simulink library "FF_Library"  (R2024b)
settings: Solver=VariableStepAuto  StartTime=0.0  StopTime=10.0  RelTol=1e-3
undefined symbols (not defined in the file or in its folder): Slope1, Slope2
libraries: simulink x60
(part 4 of 4)

== system FF_Library/Memory/SAMPLEANDHOLD_RE/Functionality ==
  u : Inport
  E : Inport  Port=2
  R : Inport  Port=3
  IV : Inport  Port=4
  x_in : Inport  Port=5
  Data Type Duplicate : DataTypeDuplicate  NumInputPorts=3
  Signal Conversion : SignalConversion  ConversionOutput=Contiguous copy  OverrideOpt=off
  Signal Conversion1 : SignalConversion  ConversionOutput=Contiguous copy  OverrideOpt=off
  Switch : Switch  Criteria=u2 ~= 0  OutDataTypeStr=Inherit: Inherit via back propagation  SaturateOnIntegerOverflow=off
  Switch1 : Switch  Criteria=u2 ~= 0  OutDataTypeStr=Inherit: Inherit via back propagation  SaturateOnIntegerOverflow=off
  y : Outport
  x_out : Outport  Port=2
  wires:
  Switch/1 -> Data Type Duplicate/1, Signal Conversion1/1, Signal Conversion/1
  x_in/1 -> Data Type Duplicate/2, Switch1/3
  u/1 -> Switch1/1
  E/1 -> Switch1/2
  Switch1/1 -> Switch/3
  IV/1 -> Data Type Duplicate/3, Switch/1
  R/1 -> Switch/2
  Signal Conversion/1 -> y/1
  Signal Conversion1/1 -> x_out/1

== system FF_Library/Ctrl/PID/PID/Delay_Ext_Reset_IV ==
  u : Inport
  R : Inport  Port=2  OutDataTypeStr=boolean
  IV : Inport  Port=3
  Constant : Constant  Value=0  OutDataTypeStr=boolean
  Data Type Duplicate : DataTypeDuplicate  NumInputPorts=3
  OR : Logic  Operator=OR  OutDataTypeStr=boolean
  Switch2 : Switch  Criteria=u2 > Threshold  InputSameDT=off
      settings: AttributesFormatString=%<Criteria>
  Unit Delay : UnitDelay  SampleTime=-1  HasFrameUpgradeWarning=on
      settings: AttributesFormatString=%<InitialCondition>
  Unit Delay1 : UnitDelay  InitialCondition=1  SampleTime=-1  HasFrameUpgradeWarning=on
      settings: AttributesFormatString=%<InitialCondition>
  y : Outport
  wires:
  Switch2/1 -> y/1, Data Type Duplicate/1
  u/1 -> Unit Delay/1, Data Type Duplicate/3
  R/1 -> OR/1
  Constant/1 -> Unit Delay1/1
  Unit Delay/1 -> Switch2/3
  IV/1 -> Switch2/1, Data Type Duplicate/2
  Unit Delay1/1 -> OR/2
  OR/1 -> Switch2/2

== system FF_Library/Ctrl/PID/PID/Delay_Ext_Reset_IV1 ==
  u : Inport
  R : Inport  Port=2  OutDataTypeStr=boolean
  IV : Inport  Port=3
  Constant : Constant  Value=0  OutDataTypeStr=boolean
  Data Type Duplicate : DataTypeDuplicate  NumInputPorts=3
  OR : Logic  Operator=OR  OutDataTypeStr=boolean
  Switch2 : Switch  Criteria=u2 > Threshold  InputSameDT=off
      settings: AttributesFormatString=%<Criteria>
  Unit Delay : UnitDelay  SampleTime=-1  HasFrameUpgradeWarning=on
      settings: AttributesFormatString=%<InitialCondition>
  Unit Delay1 : UnitDelay  InitialCondition=1  SampleTime=-1  HasFrameUpgradeWarning=on
      settings: AttributesFormatString=%<InitialCondition>
  y : Outport
  wires:
  Switch2/1 -> y/1, Data Type Duplicate/1
  u/1 -> Unit Delay/1, Data Type Duplicate/3
  R/1 -> OR/1
  Constant/1 -> Unit Delay1/1
  Unit Delay/1 -> Switch2/3
  IV/1 -> Switch2/1, Data Type Duplicate/2
  Unit Delay1/1 -> OR/2
  OR/1 -> Switch2/2

== system FF_Library/Filter/HIGHPASST_RE/Functionality/DIV ==
  In1 : Inport
  In2 : Inport  Port=2
  Constant2 : Constant  Value=abs(MinRange)  OutDataTypeStr=Inherit: Inherit via back propagation
  Constant3 : Constant  Value=-abs(MinRange)  OutDataTypeStr=Inherit: Inherit via back propagation
  Constant7 : Constant  Value=0  OutDataTypeStr=Inherit: Inherit via back propagation
  Divide1 : Product  Inputs=*/  SaturateOnIntegerOverflow=on
  Max2 : MinMax  Function=max  Inputs=2
  Min : MinMax  Inputs=2
  Relational Operator : RelationalOperator  OutDataTypeStr=boolean  RndMeth=Simplest  InputSameDT=off
  Switch : Switch  Criteria=u2 > Threshold  InputSameDT=off
  Out1 : Outport
  wires:
  Constant3/1 -> Min/2
  Min/1 -> Switch/3
  Constant2/1 -> Max2/2
  In1/1 -> Divide1/1
  Divide1/1 -> Out1/1
  Relational Operator/1 -> Switch/2
  Switch/1 -> Divide1/2
  Constant7/1 -> Relational Operator/2
  In2/1 -> Relational Operator/1, Max2/1, Min/1
  Max2/1 -> Switch/1

== system FF_Library/Filter/HIGHPASST_RE/Functionality/DIV1 ==
  In1 : Inport
  In2 : Inport  Port=2
  Constant2 : Constant  Value=abs(MinRange)  OutDataTypeStr=Inherit: Inherit via back propagation
  Constant3 : Constant  Value=-abs(MinRange)  OutDataTypeStr=Inherit: Inherit via back propagation
  Constant7 : Constant  Value=0  OutDataTypeStr=Inherit: Inherit via back propagation
  Divide1 : Product  Inputs=*/  SaturateOnIntegerOverflow=on
  Max2 : MinMax  Function=max  Inputs=2
  Min : MinMax  Inputs=2
  Relational Operator : RelationalOperator  OutDataTypeStr=boolean  RndMeth=Simplest  InputSameDT=off
  Switch : Switch  Criteria=u2 > Threshold  InputSameDT=off
  Out1 : Outport
  wires:
  Max2/1 -> Switch/1
  In2/1 -> Min/1, Max2/1, Relational Operator/1
  Constant7/1 -> Relational Operator/2
  Switch/1 -> Divide1/2
  Relational Operator/1 -> Switch/2
  Divide1/1 -> Out1/1
  In1/1 -> Divide1/1
  Constant2/1 -> Max2/2
  Min/1 -> Switch/3
  Constant3/1 -> Min/2

== system FF_Library/Limit/GRADIENTLIMITER/Functionality/Subfunctionality ==
  LUdT : Inport
  LDdT : Inport  Port=2
  x_in : Inport  Port=3
  diff_ux : Inport  Port=4
  u : Inport  Port=5
  IV : Inport  Port=6
  R : Inport  Port=7
  E : Inport  Port=8
  Add : Sum
  Add1 : Sum
  Constant4 : Constant  Value=0  OutDataTypeStr=Inherit: Inherit via back propagation
  Relational Operator : RelationalOperator  Operator=>  OutDataTypeStr=float('double')  InputSameDT=off
  Relational Operator1 : RelationalOperator  Operator=<  OutDataTypeStr=float('double')  InputSameDT=off
  Switch{2..3,6..7} (4 alike) : Switch  Criteria=u2 ~= 0  OutDataTypeStr=Inherit: Inherit via back propagation  SaturateOnIntegerOverflow=off
  Switch5 : Switch  Criteria=u2 ~= 0  SaturateOnIntegerOverflow=off
  Bmax : Outport
  Bmin : Outport  Port=2
  x_out : Outport  Port=3
  wires:
  LDdT/1 -> Add1/1, Relational Operator1/2
  LUdT/1 -> Add/1, Relational Operator/2
  Switch7/1 -> Bmin/1
  Constant4/1 -> Switch7/1
  Relational Operator/1 -> Switch7/2, Switch5/2, Bmax/1
  Relational Operator1/1 -> Switch6/2, Switch7/3
  diff_ux/1 -> Relational Operator/1, Relational Operator1/1
  R/1 -> Switch2/2
  IV/1 -> Switch2/1
  Switch3/1 -> Switch2/3
  Switch2/1 -> x_out/1
  E/1 -> Switch3/2
  Add/1 -> Switch5/1
  Add1/1 -> Switch6/1
  Switch5/1 -> Switch3/1
  Switch6/1 -> Switch5/3
  x_in/1 -> Add/2, Add1/2, Switch3/3
  u/1 -> Switch6/3

== stateflow chart FF_Library/Memory/SlideMemory/Chart1 ==
  (default) -> (junction 20) : {A=Y;}
  (junction 20) -> (junction 3) [order 1] : [En==1]{index=0;}
  (junction 3) -> (junction 5) [order 1] : [index<num-1]
  (junction 9) -> (junction 3)
  (junction 20) -> (junction 23) [order 2]
  (junction 3) -> (junction 12) [order 2] : {A[num-1]=X;}
  (junction 5) -> (junction 9) : {A[index]=A[index+1];index=index+1;}
  (junction 12) -> (junction 23)
  data: Y input; A output single; index local uint8 size=1; X input; En input; num input single size=1

== stateflow chart FF_Library/Base/Flip_Unit16HighAndLowBit/Chart4 ==
  (default) -> (junction 46)
  (junction 46) -> (junction 38) : {
      | Out_Uint16=0;
      | Out_Uint16=((In_Uint16&65280)>>8)|((In_Uint16&255)<<8);
      | }
  data: In_Uint16 input uint16; Out_Uint16 output uint16

== stateflow chart FF_Library/Filter/Moving_Average/Moving Average ==
  (default) -> (junction 1)
  (junction 1) -> (junction 12) [order 1] : [Reset]
  (junction 1) -> (junction 2) [order 2]
  (junction 12) -> (junction 41) : {count=UINT8_ZERO;
      | sum=SINGLE_ZERO;
      | index=UINT8_ZERO;
      | array=SINGLE_ZERO;}
  (junction 2) -> (junction 4) [order 1] : [count>=arraysize]
  (junction 2) -> (junction 9) [order 2] : {count=count+UINT8_ONE;}
  (junction 4) -> (junction 7) : {sum=sum-array[index];}
  (junction 7) -> (junction 9)
  (junction 9) -> (junction 14) : {sum=sum+u;...
      | array[index]=u;...
      | average=sum/count;}
  (junction 41) -> (junction 23) : {average=InitialValue;}
  (junction 14) -> (junction 15) [order 1] : [index>=(arraysize-UINT8_ONE)]
  (junction 14) -> (junction 20) [order 2] : {index=index+UINT8_ONE;}
  (junction 15) -> (junction 18) : {index=UINT8_ZERO;}
  (junction 18) -> (junction 20)
  (junction 23) -> (junction 18)
  data: u input single; Reset input boolean; arraysize parameter uint8; count local uint8; sum local single; index local uint8; UINT8_ONE constant uint8 =1; array local single size=arraysize; UINT8_ZERO constant uint8 =0; SINGLE_ZERO constant single =0; average output single; InitialValue input single

== stateflow chart FF_Library/Base/Merge_Uint8ToUint16/Chart4 ==
  (default) -> (junction 46)
  (junction 46) -> (junction 38) : {
      | Out_Uint16=0;
      | Out_Uint16=Out_Uint16|uint16(In_Uint8_2);
      | Out_Uint16=Out_Uint16<<8;
      | Out_Uint16=Out_Uint16|uint16(In_Uint8_1);
      | }
  data: In_Uint8_1 input uint8; Out_Uint16 output uint16; In_Uint8_2 input uint8

== stateflow chart FF_Library/Counter&Timer/CounterCycle_SourceZero/Chart ==
  state Counter_NoRstNoInit
    (default) -> (junction 2) : {Cnt=InitValue;
        | EnableFlg=false;}
    Counter_NoRstNoInit -> (junction 2)
    (junction 2) -> (junction 4) [order 1] : [Enable==true]
    (junction 4) -> (junction 47) [order 1] : [EnableFlg==false]
    (junction 2) -> (junction 12) [order 2] : {Cnt=InitValue;
        | EnableFlg=false;}
    (junction 4) -> (junction 5) [order 2] : {Cnt++;}
    (junction 47) -> (junction 49) : {EnableFlg=true;}
    (junction 5) -> (junction 23) [order 1] : [Cnt>=CounterCycle]
    (junction 5) -> (junction 28) [order 2]
    (junction 23) -> (junction 25) : {Cnt=InitValue;}
    (junction 28) -> (junction 12)
    (junction 25) -> (junction 28)
    (junction 49) -> (junction 25)
    (junction 12) -> (junction 15)
  (default) -> Counter_NoRstNoInit
  data: Enable input boolean; InitValue input; CounterCycle input; Cnt output; EnableFlg local boolean
